simulink model "MATLAB_function_dynamic_system"  (R2020b)
settings: Solver=VariableStepAuto  StartTime=0.0  StopTime=10.0  RelTol=1e-3
undefined symbols (not defined in the file or in its folder): x0
settings Model: Creator=maam  LastModifiedBy=maam

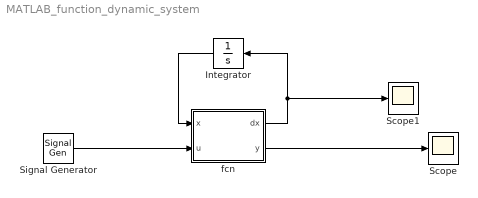
== system MATLAB_function_dynamic_system ==
  Integrator : Integrator  InitialCondition=x0
  Scope : Scope
  Scope1 : Scope
  Signal Generator : SignalGenerator  Units=rad/sec
  fcn : MATLAB Function  TreatAsAtomicUnit=on
  wires:
  Signal Generator/1 -> fcn/2(u)
  fcn/2(y) -> Scope/1
  fcn/1(dx) -> Scope1/1, Integrator/1
  Integrator/1 -> fcn/1(x)

== matlab function MATLAB_function_dynamic_system/fcn ==
  data: x input; dx output; u input; y output; p parameter
function [dx, y] = fcn(x, u, p)

    % System dynamics
    dx = zeros(size(x));
    dx(1) = x(2);
    dx(2) = -p(2) / p(1) * u;

    % System output
    y = x(1);
end
